simulink model "qbot_platform_line_follower"  (R2023a)
settings: Solver=ode1  StartTime=0.0  StopTime=inf  FixedStep=1/30  RelTol=1e-3  EnableMultiTasking=on
model workspace (MAT data in the model file):
  downCamStepSize = Simulink.Parameter
  downCamStepSize.Value = Simulink.data.Expression
  downCamStepSize.Value.ExpressionString = "qc_get_step_size*ceil(1/30/qc_get_step_size)"
  downCamStepSize.DataType = 'auto'
  downCamStepSize.Complexity = 'real'
  downCamStepSize.Dimensions = -1
  lidarStepSize = Simulink.Parameter
  lidarStepSize.Value = Simulink.data.Expression
  lidarStepSize.Value.ExpressionString = "qc_get_step_size*ceil(1/5/qc_get_step_size)"
  lidarStepSize.DataType = 'auto'
  lidarStepSize.Complexity = 'real'
  lidarStepSize.Dimensions = -1
  mainStepSize = Simulink.Parameter
  mainStepSize.Value = Simulink.data.Expression
  mainStepSize.Value.ExpressionString = "qc_get_step_size"
  mainStepSize.DataType = 'auto'
  mainStepSize.Complexity = 'real'
  mainStepSize.Dimensions = -1
  realSenseStepSize = Simulink.Parameter
  realSenseStepSize.Value = Simulink.data.Expression
  realSenseStepSize.Value.ExpressionString = "qc_get_step_size*ceil(1/30/qc_get_step_size)"
  realSenseStepSize.DataType = 'auto'
  realSenseStepSize.Complexity = 'real'
  realSenseStepSize.Dimensions = -1
undefined symbols (not defined in the file): gcbh, JPEG, video_display_show
libraries: quarc_library x20
settings Model: SimulationMode=external  ExtModeTrigDuration=10000  Creator=mbohra  LastModifiedBy=mbohra
settings SolverCC: AlgebraicLoopSolver=TrustRegion  PositivePriorityOrder=on
settings DataIOCC: ReturnWorkspaceOutputs=off
settings DebuggingCC: UnconnectedInputMsg=warning  UnconnectedOutputMsg=warning  UnconnectedLineMsg=warning  ArithmeticOperatorsInVariantConditions=warning
settings HardwareCC: ProdBitPerLong=64  ProdLargestAtomicInteger=LongLong  ProdLargestAtomicFloat=Double  ProdLongLongMode=on  ProdHWDeviceType=ARM Compatible->ARM 64-bit (LP64)
settings ModelReferenceCC: EnableRefExpFcnMdlSchedulingChecks=on
settings SFSimCC: SimUseLocalCustomCode=off  CustomCodeUndefinedFunction=UseInterfaceOnly
settings RTWCC: Description=QUARC Linux Raspberry Pi Arm64 Target (QBot Platform Alpha) Using Toolchain  SystemTargetFile=quarc_linux_pi_arm64.tlc  TemplateMakefile=quarc_default_tmf  RTWUseLocalCustomCode=off  Toolchain=QUARC linux_pi_arm64 | gmake (64-bit Windows)  BuildConfiguration=Faster Runs
settings CodeAppCC: StateflowObjectComments=on
settings STFCustomTargetCC: SystemTargetFile=quarc_linux_pi_arm64.tlc
settings GRTTargetCC: ParMdlRefBuildCompliant=off  CompOptLevelCompliant=off  CombineOutputUpdateFcns=off  MatFileLogging=off  CPPClassGenCompliant=off  GRTInterface=on  ExtMode=on  ExtModeMexFile=quarc_comm  ExtModeMexArgs='-w -d /tmp -uri %u','tcpip://192.168.2.80:17001'
settings ConfigComp: CovMetricSettings=dswe

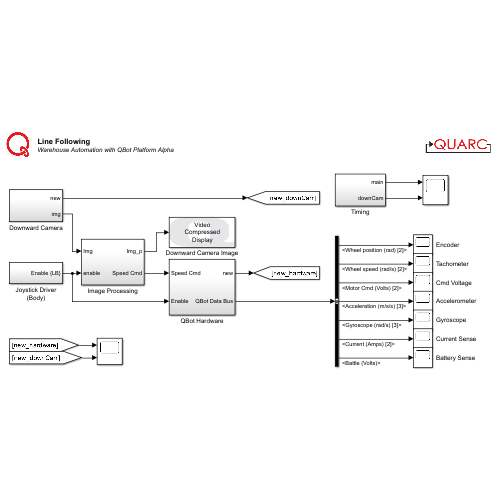
[thumbnail: Simulink's stored preview of the top-level diagram]
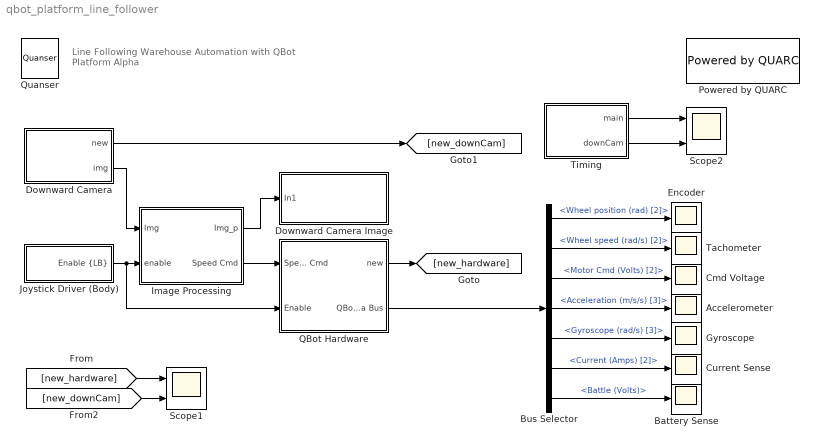
== system qbot_platform_line_follower ==
  note: Line Following
      | Warehouse Automation with QBot Platform Alpha
  Accelerometer : Scope
  Battery Sense : Scope
  Bus Selector : BusSelector  OutputSignals=Wheel position (rad) [2],Wheel speed (rad/s) [2],Motor Cmd (Volts) [2],Acceleration (m/s/s) [3],Gyroscope (rad/s) [3],Current (Amps) [2],Battle (Volts)
  Cmd Voltage : Scope
  Current Sense : Scope
  Downward Camera : Subsystem
  Downward Camera Image : Subsystem  LoadFcn=set_param(gcbh, 'UserData', gcb);  StartFcn=video_display_show([gcb, '/Video Display'], 'add', gcb);  mask(Video Compressed Display){algorithm=JPEG, quality=50, sample_time=-1, use_hardware=on}
      mask prompts: algorithm "Compression algorithm:"; quality "Compression quality (0-100):"; sample_time "Sample time (seconds):"; use_hardware "Use hardware acceleration for video display"
      mask help: Displays a video stream on the host, using compression to minimize bandwidth.
      mask init:
      | qc_set_display('Video\nCompressed\nDisplay');
      settings: UndoDeleteFcn=set_param(gcbh, 'UserData', gcb);  OpenFcn=video_display_show([gcb, '/Video Display'], 'show', gcb);  PreDeleteFcn=video_display_show([gcb, '/Video Display'], 'delete');
      settings: CopyFcn=|
      | set_param(gcbh, 'UserData', gcb);
      | set_param(gcbh, 'LinkStatus', 'none');
      settings: NameChangeFcn=|
      | video_display_show([get_param(gcbh, 'UserData'), '/Video Display'], 'rename', [gcb, '/Video Display']);
      | video_display_show([gcb, '/Video Display'], 'add', gcb);
      | set_param(gcbh, 'UserData', gcb);
      mask Help: web(qc_get_block_help_path(gcb));
      mask TypeOptions algorithm: Image Compress/algorithm
      mask TypeOptions quality: Image Compress/quality
      mask TypeOptions sample_time: Video Display/sample_time
      mask TypeOptions use_hardware: Video Display/use_hardware
      mask Display:
      | patch([0.98591 0.98591 0.62618 0.59072 0.56147   0.536   0.536  0.5441 0.56912 0.59207 0.60881 0.62276 0.63527 0.64364  0.6485  0.6485 0.64706 0.64499 0.63662 0.62411 0.61232 0.59837 0.58307 0.56147   0.536   0.536  0.5441  0.5747 0.60953 0.63662 0.67001  0.7034 0.72851 0.75425 0.77927 0.80294 0.82454 0.84119 0.85865 0.87395 0.88574 0.89339  0.8969 0.89969 0.89969 0.89267  0.8816 0.87044 0.85649  0.8384 0.81824 0.80294 0.78764 0.77513 0.76676 0.75776 0.76397 0.77513 0.79178 0.80987 0.82796 0.84326 0.86207 0.98528],[0.18689 0.05522 0.05522 0.05171 0.05171    0.05 0.18338 0.18338 0.19148 0.20435 0.22298 0.24863 0.28589 0.33125 0.38138 0.55139 0.59801 0.63761 0.68189 0.72149 0.74939 0.76694 0.77855 0.79367 0.79952 0.92768 0.92768 0.92768 0.92417 0.92066 0.91364  0.9032 0.89384 0.88106 0.86594 0.85073 0.82634 0.80537 0.77855 0.74363 0.70403 0.65858 0.61079 0.59099 0.41513 0.37202 0.31847 0.29048 0.25556 0.23342  0.2102 0.19382 0.18221 0.17285 0.16943 0.16124  0.1589 0.16241 0.16709 0.17168  0.1787 0.18221 0.18689 0.18689],[0.9,0.90,0.91])
      | patch([0.536 0.52601 0.46823 0.44528 0.41603 0.39101 0.35555 0.33116 0.31451 0.29291  0.2804 0.26717 0.25322 0.23999 0.22406 0.20732 0.19337 0.17528 0.15935 0.14396 0.13217 0.11759 0.10922 0.10085 0.09671 0.09392 0.09041 0.08906 0.08906 0.09464  0.0995 0.10778 0.11894 0.13145 0.14675 0.16349 0.17672 0.19409 0.20732 0.22406 0.23999 0.26159 0.27833 0.29849 0.31793 0.33602 0.35411 0.37085 0.39245 0.41603   0.536   0.536 0.53159 0.46409   0.446 0.42026 0.39587 0.37571 0.36113 0.34925 0.34088 0.33809 0.33809 0.34088 0.34583 0.35627 0.36392 0.38129 0.39587 0.41117 0.42719 0.44672  0.4676 0.48353 0.48353 0.52394   0.536],[0.05 0.04829 0.04712 0.04712 0.04829 0.05063 0.05405 0.05873 0.06107 0.06692 0.07043 0.07619 0.08087 0.08672 0.09482 0.10652 0.11696 0.13325  0.1508 0.17168 0.19499 0.22415 0.25439 0.28472 0.31379 0.35456 0.38489 0.41513 0.58055 0.63878 0.68774 0.72149 0.75641 0.78089 0.80537 0.82859 0.84029 0.85658 0.86594 0.87404  0.8834 0.89267 0.90086 0.90788 0.91247 0.91832 0.92066   0.923 0.92651 0.92768 0.92768 0.79952 0.79952 0.79952 0.79718 0.78899 0.77153 0.75056 0.72149 0.68072 0.62249  0.5549 0.41396 0.37085 0.33242 0.28121 0.25205 0.22181 0.20552 0.19499 0.18572 0.18221 0.17753 0.17636 0.17753  0.1787  0.1787],[0.9,0.90,0.91])
      | disp('Video\nCompressed\nDisplay');
  Encoder : Scope
  Gyroscope : Scope
  Image Processing : Subsystem
  Joystick Driver (Body) : Subsystem
  Powered by QUARC : quarc_library/Logos/Powered by QUARC
  QBot Hardware : Subsystem
  Quanser : quarc_library/Logos/Quanser
  Scope1 : Scope  NumInputPorts=2
  Scope2 : Scope  NumInputPorts=2
  Tachometer : Scope
  Timing : Subsystem
  wires:
  Timing/1(main) -> Scope2/1
  Timing/2(downCam) -> Scope2/2
  QBot Hardware/2(QBot Data Bus) -> Bus Selector/1
  QBot Hardware/1(new) -> [new_hardware]
  Downward Camera/1(new) -> [new_downCam]
  [new_hardware] -> Scope1/1
  [new_downCam] -> Scope1/2
  Bus Selector/1 -> Encoder/1  "<Wheel position (rad) [2]>"
  Bus Selector/3 -> Cmd Voltage/1  "<Motor Cmd (Volts) [2]>"
  Bus Selector/4 -> Accelerometer/1  "<Acceleration (m/s/s) [3]>"
  Bus Selector/6 -> Current Sense/1  "<Current (Amps) [2]>"
  Bus Selector/2 -> Tachometer/1  "<Wheel speed (rad/s) [2]>"
  Bus Selector/5 -> Gyroscope/1  "<Gyroscope (rad/s) [3]>"
  Bus Selector/7 -> Battery Sense/1  "<Battle (Volts)>"
  Downward Camera/2(img) -> Image Processing/1(Img)
  Image Processing/2(Speed Cmd) -> QBot Hardware/1(Speed Cmd)
  Joystick Driver (Body)/1("Enable {LB}") -> Image Processing/2(enable), QBot Hardware/2(Enable)
  Image Processing/1(Img_p) -> Downward Camera Image/1(In1)

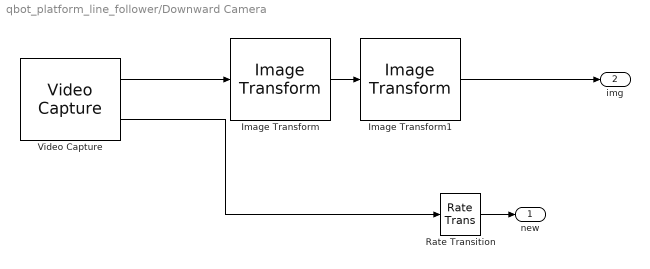
== system qbot_platform_line_follower/Downward Camera ==
  Image Transform : quarc_library/Image Processing/Generic/Image Transform  algorithm=Lens undistort  color_theme=KRYGCBMW  min_pixel=0  max_pixel=4000  focal_length=[302.1629, 301.7493]  principal_point=[185.6271, 306.7551]  radial_coeffs=[-0.3138 0.0780]  tangential_coeffs=[]  extrapolated_pixel=0  interpolation=nearest  row_coords=0  column_coords=0  output_height=480  output_width=640  angle=0  origin=[240 320]  output_origin=[240 320]  output_data_type=uint8
      settings: AttributesFormatString=(%<algorithm>)  SourceProductName=QUARC Targets
  Image Transform1 : quarc_library/Image Processing/Generic/Image Transform  algorithm=Resize  color_theme=KRYGCBMW  min_pixel=0  max_pixel=4000  focal_length=308  principal_point=[262 334]  radial_coeffs=[-0.3129 0.0907]  tangential_coeffs=[]  extrapolated_pixel=0  interpolation=nearest  row_coords=0  column_coords=0  output_height=200  output_width=320  angle=0  origin=[240 320]  output_origin=[240 320]  output_data_type=uint8
      settings: AttributesFormatString=(%<algorithm>)  SourceProductName=QUARC Targets
  Rate Transition : RateTransition
  Video Capture : quarc_library/Multimedia/Video Capture  source=device  device=6  filename=sample_movie.mov  value=[0 0; 0 0]  resolution=640 x 400  width=640  height=400  output_format=MATLAB greyscale (HxW)  data_type=uint8  sample_time=downCamStepSize  brightness_override=off  brightness=50.0  contrast_override=off  contrast=50.0  hue_override=off  hue=50.0  saturation_override=off  saturation=50.0  sharpness_override=off  sharpness=50.0  gamma_override=off  gamma=50.0  coloreffect_override=off  coloreffect=None  whitebalance_override=off  whitebalance=50.0  backlightcompensation_override=off  backlightcompensation=0.0  gain_override=on  gain=17.0  pan_override=off  pan=50.0  tilt_override=off  tilt=50.0  roll_override=off  roll=50.0  zoom_override=off  zoom=0.0  exposure_override=on  exposure=39.0  iris_override=off  iris=50.0  mirror_override=off  mirror=None  focus_override=off  focus=0.0
      settings: SourceProductName=QUARC Targets
  new : Outport
  img : Outport  Port=2
  wires:
  Video Capture/2 -> Rate Transition/1
  Image Transform1/1 -> img/1
  Rate Transition/1 -> new/1
  Video Capture/1 -> Image Transform/1
  Image Transform/1 -> Image Transform1/1

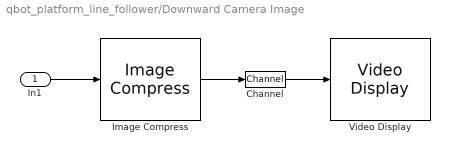
== system qbot_platform_line_follower/Downward Camera Image ==
  In1 : Inport
  Channel : quarc_library/Signal Routing/Channel  channel=0  buffer_size=1
  Image Compress : quarc_library/Image Processing/Generic/Image Compress  algorithm=JPEG  source=Internal dialog parameter  quality=quality  output_dim=-1
  Video Display : quarc_library/Multimedia/Video Display  Tag=qbot_platform_line_follower/Downward Camera Image/Video Display  sample_time=sample_time  use_hardware=on
  wires:
  Channel/1 -> Video Display/1
  In1/1 -> Image Compress/1
  Image Compress/1 -> Channel/1

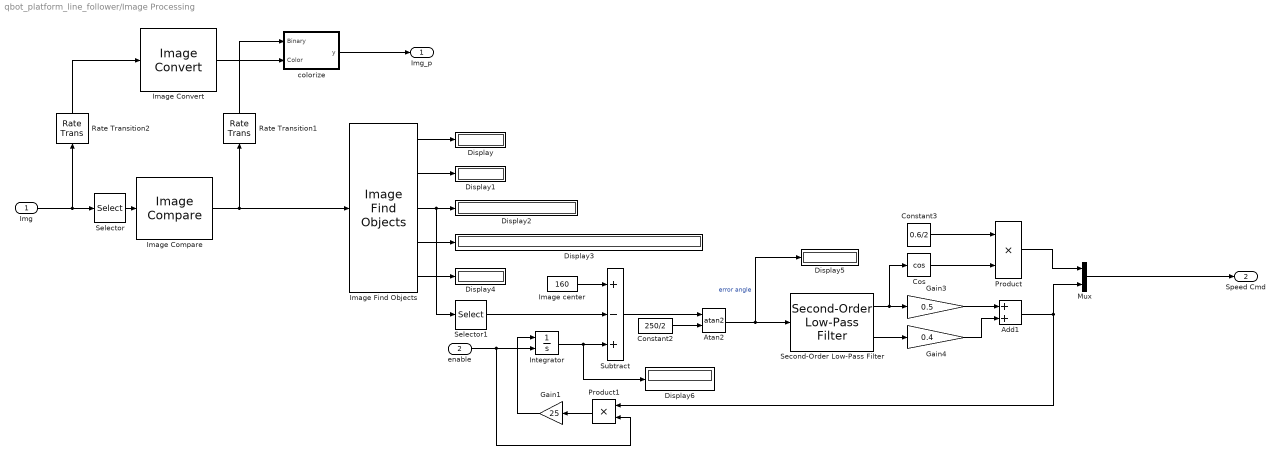
== system qbot_platform_line_follower/Image Processing ==
  Img : Inport
  enable : Inport  Port=2
  Add1 : Sum
  Atan2 : Trigonometry  Operator=atan2
  Constant2 : Constant  Value=250/2
  Constant3 : Constant  Value=0.6/2
  Cos : Trigonometry  Operator=cos
  Display{,1..6} (7 alike) : Display
      Display settings: Format=bank
      Display1 settings: Format=bank
      Display2 settings: Format=bank
      Display3 settings: Format=bank
      Display4 settings: Format=bank
  Gain1 : Gain  Gain=25
  Gain3 : Gain  Gain=0.5
  Gain4 : Gain  Gain=0.4
  Image Compare : quarc_library/Image Processing/Generic/Image Compare  output_type=Combined (one HxW output)  source=Internal dialog parameters  r_comparison=min <= pixel and pixel <= max  r_minimum=225  r_maximum=255  g_comparison=min <= pixel and pixel <= max  g_minimum=225  g_maximum=255  b_comparison=min <= pixel and pixel <= max  b_minimum=225  b_maximum=255
      settings: SourceProductName=QUARC Targets
  Image Convert : quarc_library/Image Processing/Generic/Image Convert  input_format=MATLAB greyscale (HxW)  padding=0  output_format=MATLAB RGB (HxWx3)  data_type=uint8
      settings: AttributesFormatString=(%<input_format>)  SourceProductName=QUARC Targets
  Image Find Objects : quarc_library/Image Processing/Generic/Image Find Objects  num_objects=1  connectivity=8 directions (N, NE, E, SE, S, SW, W, NW)  sort_order=Sort by number of pixels  min_pixels=500  max_pixels=intmax('uint32')  largest=on  exclude_at_edges=off  variable_size=off  use_complex=off
      settings: SourceProductName=QUARC Targets
  Image center : Constant  Value=160
  Integrator : Integrator  ExternalReset=falling  LimitOutput=on  UpperSaturationLimit=50  LowerSaturationLimit=-50
  Mux : Mux  Inputs=2
  Product : Product
  Product1 : Product
  Rate Transition1 : RateTransition  OutPortSampleTime=downCamStepSize*2
  Rate Transition2 : RateTransition  OutPortSampleTime=downCamStepSize*2
  Second-Order Low-Pass Filter : quarc_library/Continuous/Second-Order Low-Pass Filter  params_source=Internal (dialog parameters)  input_width=2*pi*5  input_zeta=1  input_init=0
  Selector : Selector  NumberOfDimensions=2  InputPortWidth=3  IndexOptions=Index vector (dialog),Select all  Indices=[51:100],[101:540]  OutputSizes=1,1
  Selector1 : Selector  InputPortWidth=2  IndexOptions=Index vector (dialog)  Indices=2  OutputSizes=1
  Subtract : Sum  Inputs=+-+
  colorize : MATLAB Function  TreatAsAtomicUnit=on
  Img_p : Outport
  Speed Cmd : Outport  Port=2
  wires:
  Selector1/1 -> Subtract/2
  Image center/1 -> Subtract/1
  Image Find Objects/5 -> Display4/1
  Image Find Objects/3 -> Display2/1, Selector1/1
  Image Find Objects/4 -> Display3/1
  Image Find Objects/2 -> Display1/1
  Image Find Objects/1 -> Display/1
  Image Compare/1 -> Image Find Objects/1, Rate Transition1/1
  Img/1 -> Rate Transition2/1, Selector/1
  Selector/1 -> Image Compare/1
  Rate Transition1/1 -> colorize/1(Binary)
  Atan2/1 -> Display5/1, Second-Order Low-Pass Filter/1  "error angle"
  Subtract/1 -> Atan2/1
  Constant2/1 -> Atan2/2
  Cos/1 -> Product/2
  Constant3/1 -> Product/1
  Product/1 -> Mux/1
  Mux/1 -> Speed Cmd/1
  Add1/1 -> Product1/1, Mux/2
  Integrator/1 -> Display6/1, Subtract/3
  Gain1/1 -> Integrator/1
  enable/1 -> Product1/2, Integrator/2
  Gain4/1 -> Add1/2
  Gain3/1 -> Add1/1
  Second-Order Low-Pass Filter/2 -> Gain4/1
  Second-Order Low-Pass Filter/1 -> Cos/1, Gain3/1
  Product1/1 -> Gain1/1
  Rate Transition2/1 -> Image Convert/1
  colorize/1(y) -> Img_p/1
  Image Convert/1 -> colorize/2(Color)

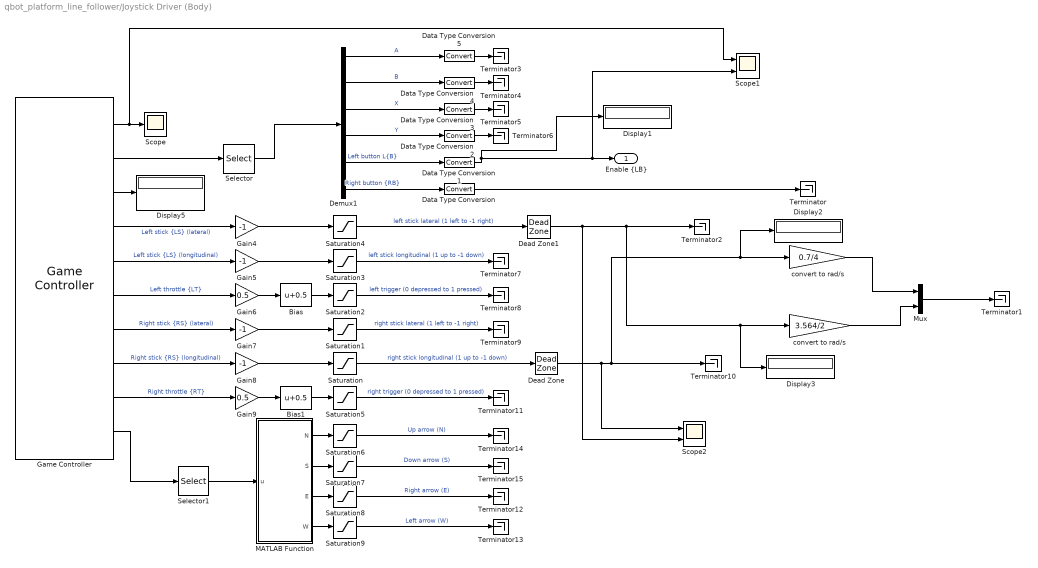
== system qbot_platform_line_follower/Joystick Driver (Body) ==
  Bias : Bias  Bias=0.5  SaturateOnIntegerOverflow=off
  Bias1 : Bias  Bias=0.5  SaturateOnIntegerOverflow=off
  Data Type Conversion{,1..5} (6 alike) : DataTypeConversion  SaturateOnIntegerOverflow=off  RndMeth=Floor
  Dead Zone : DeadZone  LowerValue=-0.05  UpperValue=0.05
  Dead Zone1 : DeadZone  LowerValue=-0.05  UpperValue=0.05
  Demux1 : Demux  Outputs=6
  Display{1..3,5} (4 alike) : Display
  Gain{4..5,7..8} (4 alike) : Gain  Gain=-1
  Gain6 : Gain  Gain=0.5
  Gain9 : Gain  Gain=0.5
  Game Controller : quarc_library/Devices/Peripherals/Target/Game Controller  controller=1  buffer_size=12  deadzone=[]  saturation=[]  sample_time=qc_get_step_size  auto_center=off  enabled=on
      settings: SourceProductName=QUARC Targets
  MATLAB Function : MATLAB Function  TreatAsAtomicUnit=on
  Mux : Mux  Inputs=2
  Saturation{,1,3..4} (4 alike) : Saturate  UpperLimit=1  LowerLimit=-1
  Saturation{2,5..9} (6 alike) : Saturate  UpperLimit=1  LowerLimit=0
  Scope : Scope
  Scope1 : Scope  NumInputPorts=2
  Scope2 : Scope  NumInputPorts=2
  Selector : Selector  InputPortWidth=32  IndexOptions=Index vector (dialog)  Indices=[1:6]  OutputSizes=1
  Selector1 : Selector  InputPortWidth=4  IndexOptions=Index vector (dialog)  Indices=1  OutputSizes=1
  Terminator{,1..15} (16 alike) : Terminator
  convert to rad/s : Gain  Gain=0.7/4
  "convert to rad/s " : Gain  Gain=3.564/2
  "Enable {LB}" : Outport
  wires:
  convert to rad/s/1 -> Mux/1
  Mux/1 -> Terminator1/1
  Game Controller/1 -> Scope1/1, Scope/1
  Game Controller/2 -> Selector/1
  Game Controller/3 -> Display5/1
  Game Controller/4 -> Gain4/1  "Left stick {LS} (lateral)"
  Game Controller/5 -> Gain5/1  "Left stick {LS} (longitudinal)"
  Game Controller/6 -> Gain6/1  "Left throttle {LT}"
  Game Controller/7 -> Gain7/1  "Right stick {RS} (lateral)"
  Game Controller/8 -> Gain8/1  "Right stick {RS} (longitudinal)"
  Game Controller/9 -> Gain9/1  "Right throttle {RT}"
  Game Controller/10 -> Selector1/1
  Selector/1 -> Demux1/1
  Demux1/1 -> Data Type Conversion5/1  "A"
  Demux1/2 -> Data Type Conversion4/1  "B"
  Demux1/3 -> Data Type Conversion3/1  "X"
  Demux1/4 -> Data Type Conversion2/1  "Y"
  Demux1/5 -> Data Type Conversion1/1  "Left button L{B}"
  Demux1/6 -> Data Type Conversion/1  "Right button {RB}"
  Selector1/1 -> MATLAB Function/1(u)
  Gain6/1 -> Bias/1
  Gain9/1 -> Bias1/1
  Gain8/1 -> Saturation/1
  Gain7/1 -> Saturation1/1
  Gain5/1 -> Saturation3/1
  Gain4/1 -> Saturation4/1
  Bias/1 -> Saturation2/1
  Bias1/1 -> Saturation5/1
  Saturation4/1 -> Dead Zone1/1  "left stick lateral (1 left to -1 right)"
  Saturation3/1 -> Terminator7/1  "left stick longitudinal (1 up to -1 down)"
  Saturation2/1 -> Terminator8/1  "left trigger (0 depressed to 1 pressed)"
  Saturation1/1 -> Terminator9/1  "right stick lateral (1 left to -1 right)"
  Saturation/1 -> Dead Zone/1  "right stick longitudinal (1 up to -1 down)"
  Saturation5/1 -> Terminator11/1  "right trigger (0 depressed to 1 pressed)"
  MATLAB Function/1(N) -> Saturation6/1
  MATLAB Function/2(S) -> Saturation7/1
  MATLAB Function/3(E) -> Saturation8/1
  MATLAB Function/4(W) -> Saturation9/1
  Saturation6/1 -> Terminator14/1  "Up arrow (N)"
  Saturation7/1 -> Terminator15/1  "Down arrow (S)"
  Saturation8/1 -> Terminator12/1  "Right arrow (E)"
  Saturation9/1 -> Terminator13/1  "Left arrow (W)"
  Data Type Conversion1/1 -> Display1/1, Scope1/2, "Enable {LB}"/1
  Data Type Conversion2/1 -> Terminator6/1
  Data Type Conversion3/1 -> Terminator5/1
  Data Type Conversion4/1 -> Terminator4/1
  Data Type Conversion5/1 -> Terminator3/1
  Data Type Conversion/1 -> Terminator/1
  "convert to rad/s "/1 -> Mux/2
  Dead Zone/1 -> Scope2/1, convert to rad/s/1, Display2/1, Terminator10/1
  Dead Zone1/1 -> Scope2/2, "convert to rad/s "/1, Display3/1, Terminator2/1

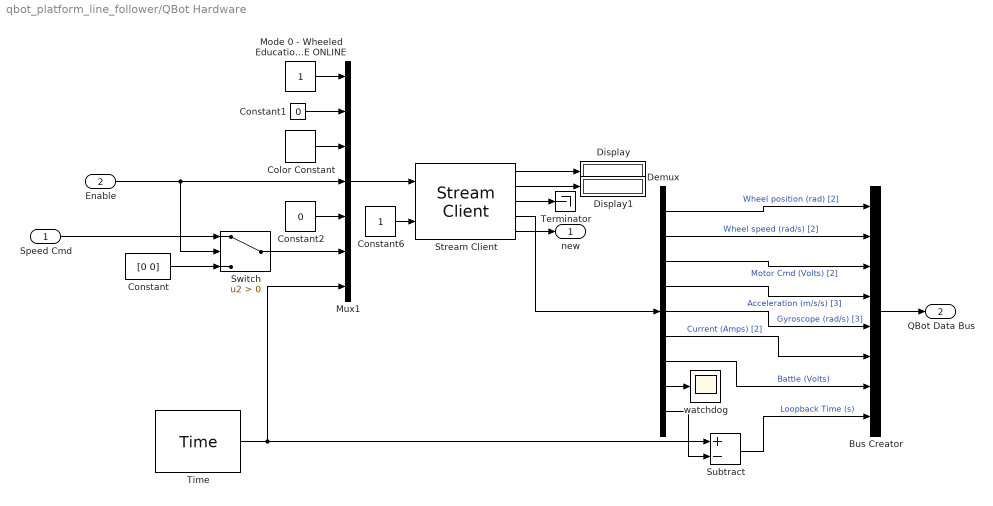
== system qbot_platform_line_follower/QBot Hardware ==
  Speed Cmd : Inport
  Enable : Inport  Port=2
  Bus Creator : BusCreator  Inputs=8
  Color Constant : quarc_library/Sources/Signals/Color Constant  color=[0 1 1]
      settings: SourceProductName=QUARC Targets
  Constant : Constant  Value=[0 0]
  Constant1 : Constant  Value=0
  Constant2 : Constant  Value=0
  Constant6 : Constant
  Demux : Demux  Outputs=[2 2 2 3 3 2 1 1 1]
  Display : Display
  Display1 : Display
  Mode 0 - Wheeled Education Mode Mode 1 - Body Education Mode Mode 2 - Wheeled Research Mode Mode 3 - Body Research Mode DO NOT CHANGE ONLINE : Constant
  Mux1 : Mux  Inputs=7
  Stream Client : quarc_library/Communications/Basic/Stream Client  uri_source=Specify via dialog (do not evaluate)  uri=tcpip://localhost:18888  send_buffer_size=1460  receive_buffer_size=1460  byte_order=little endian (Intel - LSB first)  optimization=Minimum latency  send_options=Send most recent data  receive_options=Receive most recent data  default_value=zeros(17,1)  sample_time=qc_get_step_size  active=off  implementation=Use blocking I/O in a separate thread  send_fifo_size=1000  receive_fifo_size=1000  send_priority=0  receive_priority=0  send_dimensions=off  receive_dimensions=off  max_dimensions=-1  data_type=Inherited via back propagation  type_expr=BusObject
      settings: AttributesFormatString="\"tcpip://localhost:18888\""
  Subtract : Sum  Inputs=+-
  Switch : Switch  Criteria=u2 > Threshold  SaturateOnIntegerOverflow=off  InputSameDT=off
  Terminator : Terminator
  Time : quarc_library/Sources/Time/Time  time_source=Wall clock  sample_time=qc_get_step_size
  watchdog : Scope
  new : Outport
  QBot Data Bus : Outport  Port=2
  wires:
  Demux/2 -> Bus Creator/2  "Wheel speed (rad/s) [2]"
  Mode 0 - Wheeled Education Mode Mode 1 - Body Education Mode Mode 2 - Wheeled Research Mode Mode 3 - Body Research Mode DO NOT CHANGE ONLINE/1 -> Mux1/1
  Stream Client/3 -> Terminator/1
  Speed Cmd/1 -> Switch/1
  Stream Client/1 -> Display/1
  Constant6/1 -> Stream Client/2
  Stream Client/2 -> Display1/1
  Color Constant/1 -> Mux1/3
  Constant1/1 -> Mux1/2
  Demux/3 -> Bus Creator/3  "Motor Cmd (Volts) [2]"
  Mux1/1 -> Stream Client/1
  Stream Client/4 -> Demux/1
  Demux/1 -> Bus Creator/1  "Wheel position (rad) [2]"
  Stream Client/5 -> new/1
  Demux/7 -> Bus Creator/7  "Battle (Volts)"
  Demux/5 -> Bus Creator/5  "Gyroscope (rad/s) [3]"
  Demux/6 -> Bus Creator/6  "Current (Amps) [2]"
  Demux/9 -> Subtract/2
  Constant2/1 -> Mux1/5
  Demux/4 -> Bus Creator/4  "Acceleration (m/s/s) [3]"
  Enable/1 -> Switch/2, Mux1/4
  Time/1 -> Mux1/7, Subtract/1
  Bus Creator/1 -> QBot Data Bus/1
  Subtract/1 -> Bus Creator/8  "Loopback Time (s)"
  Demux/8 -> watchdog/1
  Switch/1 -> Mux1/6
  Constant/1 -> Switch/3

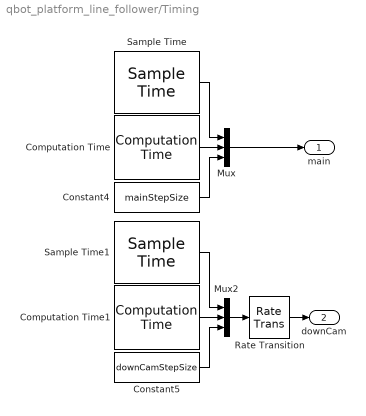
== system qbot_platform_line_follower/Timing ==
  Computation Time : quarc_library/Sources/Time/Computation Time  sample_time=mainStepSize  use_model=on  use_cpu_time=off
  Computation Time1 : quarc_library/Sources/Time/Computation Time  sample_time=downCamStepSize  use_model=on  use_cpu_time=off
  Constant4 : Constant  Value=mainStepSize
  Constant5 : Constant  Value=downCamStepSize
  Mux : Mux  Inputs=3
  Mux2 : Mux  Inputs=3
  Rate Transition : RateTransition
  Sample Time : quarc_library/Sources/Time/Sample Time  Priority=-99  sample_time=mainStepSize
  Sample Time1 : quarc_library/Sources/Time/Sample Time  Priority=-99  sample_time=downCamStepSize
  main : Outport
  downCam : Outport  Port=2
  wires:
  Constant5/1 -> Mux2/3
  Computation Time/1 -> Mux/2
  Sample Time/1 -> Mux/1
  Sample Time1/1 -> Mux2/1
  Computation Time1/1 -> Mux2/2
  Constant4/1 -> Mux/3
  Mux2/1 -> Rate Transition/1
  Rate Transition/1 -> downCam/1
  Mux/1 -> main/1

== matlab function qbot_platform_line_follower/Joystick Driver (Body)/MATLAB Function ==
  data: u input; N output; S output; E output; W output
function [N, S, E, W] = fcn(u)

N = 0;
S = 0;
E = 0;
W = 0;

switch u
    case 0
        N = 1;
    case 3.142
        S = 1;
    case 4.712
        W = 1;
    case 1.571
        E = 1;
    case 3.927
        S = 1;
        W = 1;
    case 2.356
        S = 1;
        E = 1;
    case 0.7854
        N = 1;
        E = 1;
    case 5.498
        N = 1;
        W = 1;
end

== matlab function qbot_platform_line_follower/Image Processing/colorize ==
  data: Binary input; y output; Color input
function y = fcn(Binary, Color)

y = Color;
[ROW, COL, ~] = size(y);

y(51:100, 1:COL, 1) = ((255 - Binary)/255).*Color(51:100,:,1) + (Binary).*Color(51:100, :, 1);
y(51:100, 1:COL, 2) = ((255 - Binary)/255).*Color(51:100,:,2);
y(51:100, 1:COL, 3) = ((255 - Binary)/255).*Color(51:100,:,3);
